simulink model "complete_model_DISCR"  (R2022b)
settings: Solver=FixedStepAuto  StartTime=0.0  StopTime=300.0  RelTol=1e-3
undefined symbols (not defined in the file): DiscIntNeverNeededParam
settings Model: Creator=umber  LastModifiedBy=umber
settings DataIOCC: ExternalInput=a.getElement('current')
settings OptimizationCC: OptimizeBlockIOStorage=off  OptimizeDataStoreBuffers=off  BusAssignmentInplaceUpdate=off
settings DebuggingCC: SFUnexpectedBacktrackingDiag=warning  SFNoUnconditionalDefaultTransitionDiag=warning
settings ModelReferenceCC: EnableRefExpFcnMdlSchedulingChecks=on
settings RTWCC: GenCodeOnly=on  GenerateReport=on  BuildConfiguration=Debug  LaunchReport=on
settings CodeAppCC: ForceParamTrailComments=on  MATLABSourceComments=on  EnableCustomComments=on
settings GRTTargetCC: CombineSignalStateStructs=on  SupportVariableSizeSignals=on  MultiInstanceErrorCode=Warning

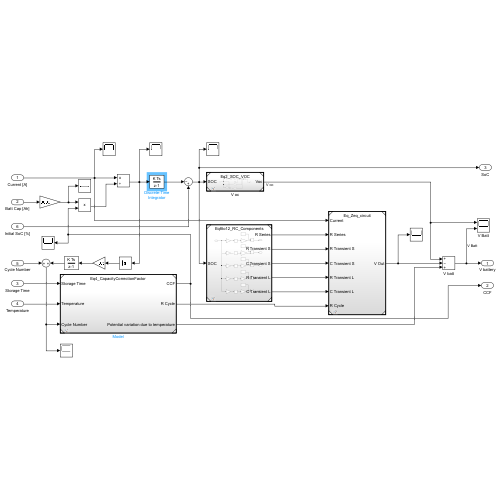
[thumbnail: Simulink's stored preview of the top-level diagram]
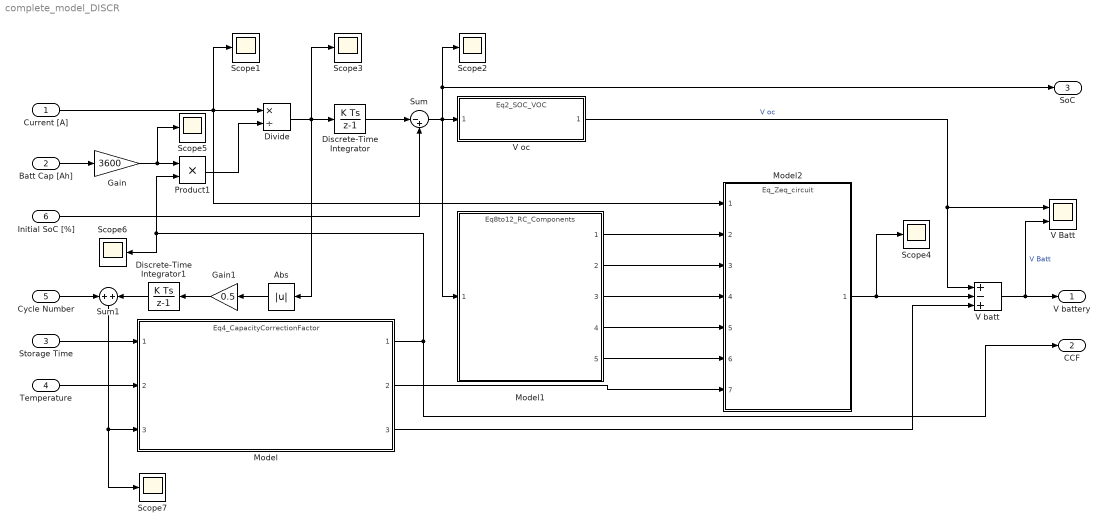
== system complete_model_DISCR ==
  Current [A] : Inport
  Batt Cap [Ah] : Inport  Port=2
  Storage Time : Inport  Port=3
  Temperature : Inport  Port=4
  Cycle Number : Inport  Port=5
  Initial SoC [%] : Inport  Port=6
  Abs : Abs  SaturateOnIntegerOverflow=off
  Discrete-Time Integrator : DiscreteIntegrator  SampleTime=-1  ICPrevOutput=DiscIntNeverNeededParam  ICPrevScaledInput=DiscIntNeverNeededParam
  Discrete-Time Integrator1 : DiscreteIntegrator  SampleTime=-1  ICPrevOutput=DiscIntNeverNeededParam  ICPrevScaledInput=DiscIntNeverNeededParam
  Divide : Product  Inputs=*/
  Gain : Gain  Gain=3600
  Gain1 : Gain  Gain=0.5
  Model : ModelReference  ModelNameDialog=Eq4_CapacityCorrectionFactor.slx  SimulationMode=Normal  ModelReferenceVersion=2.12
  Model1 : ModelReference  ModelNameDialog=Eq8to12_RC_Components  SimulationMode=Normal  ModelReferenceVersion=2.6
  Model2 : ModelReference  ModelNameDialog=Eq_Zeq_circuit.slx  SimulationMode=Normal  ModelReferenceVersion=1.16
  Product1 : Product
  Scope{1..7} (7 alike) : Scope
  Sum : Sum  Inputs=|-+
  Sum1 : Sum
  V Batt : Scope  NumInputPorts=2
  V batt : Sum  Inputs=+-+
  V oc : ModelReference  ModelNameDialog=Eq2_SOC_VOC.slx  SimulationMode=Normal  ModelReferenceVersion=2.4
  V battery : Outport
  CCF : Outport  Port=2
  SoC : Outport  Port=3
  wires:
  Divide/1 -> Discrete-Time Integrator/1, Abs/1, Scope3/1
  Discrete-Time Integrator/1 -> Sum/1
  Sum/1 -> Scope2/1, SoC/1, Model1/1, V oc/1
  Current [A]/1 -> Scope1/1, Model2/1, Divide/1
  Initial SoC [%]/1 -> Sum/2
  V oc/1 -> V batt/1, V Batt/1  "V oc"
  Model1/1 -> Model2/2
  Model/3 -> V batt/3
  Product1/1 -> Divide/2
  Batt Cap [Ah]/1 -> Gain/1
  Model2/1 -> Scope4/1, V batt/2
  Model1/2 -> Model2/3
  Model1/3 -> Model2/4
  Model1/4 -> Model2/5
  Model1/5 -> Model2/6
  Model/2 -> Model2/7
  V batt/1 -> V battery/1, V Batt/2  "V Batt"
  Storage Time/1 -> Model/1
  Temperature/1 -> Model/2
  Model/1 -> Product1/2, Scope6/1, CCF/1
  Gain/1 -> Scope5/1, Product1/1
  Gain1/1 -> Discrete-Time Integrator1/1
  Cycle Number/1 -> Sum1/1
  Discrete-Time Integrator1/1 -> Sum1/2
  Sum1/1 -> Model/3, Scope7/1
  Abs/1 -> Gain1/1
